simulink model "MIMO_FIXED"  (R2017a)
settings: Solver=VariableStepAuto  StartTime=0.0  StopTime=1000  RelTol=1e-3
libraries: dspsigops x80, commchan3 x4, commdigbbndpm3 x2, commfilt2 x2, commsink2 x1, commutil2 x1
(part 1 of 6)
settings Model: Creator=pc1  LastModifiedBy=U3
settings DataIOCC: SaveOutput=off  SignalLogging=off  DSMLogging=off  SaveTime=off
settings DebuggingCC: UnconnectedInputMsg=none  UnconnectedOutputMsg=none  UnconnectedLineMsg=none
settings SFSimCC: SimUseLocalCustomCode=on
settings RTWCC: RTWUseLocalCustomCode=on

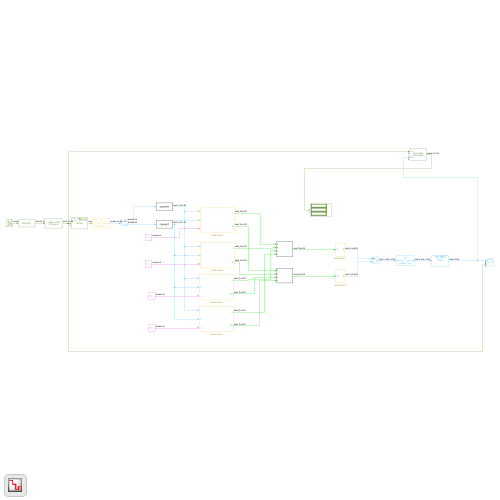
[thumbnail: Simulink's stored preview of the top-level diagram]
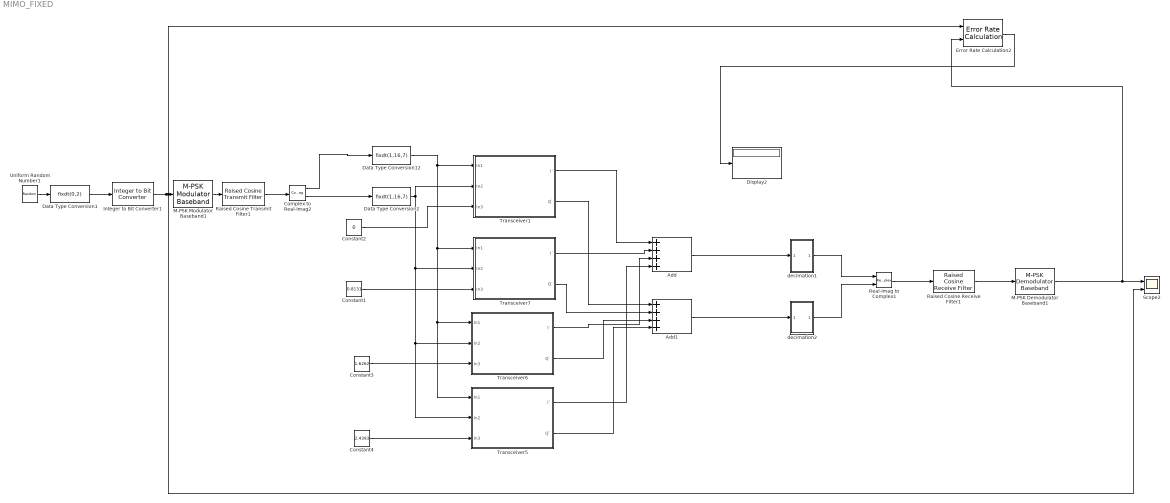
== system MIMO_FIXED ==
  Add : Sum  Inputs=++++  OutDataTypeStr=fixdt(1,8,4)
  Add1 : Sum  Inputs=++++  OutDataTypeStr=fixdt(1,8,4)
  Complex to Real-Imag2 : ComplexToRealImag
  Constant1 : Constant  Value=0.8131
  Constant2 : Constant  Value=0
  Constant3 : Constant  Value=1.6262
  Constant4 : Constant  Value=2.4393
  Data Type Conversion1 : DataTypeConversion  OutMin=0  OutMax=3  OutDataTypeStr=fixdt(0,2)  RndMeth=Round
  Data Type Conversion12 : DataTypeConversion  OutDataTypeStr=fixdt(1,16,7)  SaturateOnIntegerOverflow=on
  Data Type Conversion2 : DataTypeConversion  OutDataTypeStr=fixdt(1,16,7)  SaturateOnIntegerOverflow=on
  Display2 : Display
  Error Rate Calculation2 : commsink2/Error Rate Calculation  N=28  st_delay=0  cp_mode=Entire frame  subframe=[]  PMode=Port  WsName=ErrorVec  RsMode2=off  stop=off  numErr=100  maxBits=1e6
  Integer to Bit Converter1 : commutil2/Integer to Bit Converter  nbits=2  signedInputValues=Unsigned  bitOrder=MSB first  outDtype=Inherit via internal rule
  M-PSK Demodulator Baseband1 : commdigbbndpm3/M-PSK Demodulator Baseband  M=4  OutType=Bit  DecType=Hard decision  VarSource=Dialog  Variance=1  Dec=Gray  Mapping=[0:7]  Ph=pi/4  outDtype1=Inherit via internal rule  outDtype2=Inherit via internal rule  derotateFactorWordLen=16  derotateFactorDataTypeStr=Inherit: Same word length as input  derotateFactorLastDataTypeStr=Inherit: Same word length as input
  M-PSK Modulator Baseband1 : commdigbbndpm3/M-PSK Modulator Baseband  M=4  InType=Bit  Enc=Gray  Mapping=[0:7]  Ph=pi/4  outDtype=double  outWordLen=16  outUDDataType=sfix(16)  outFracLenMode=Best precision  outFracLen=15  outDataTypeStr=double  outLastDataTypeStr=double
  Raised Cosine Receive Filter1 : commfilt2/Raised Cosine Receive Filter  filtType=Square root  R=0.35  filtSpan=8  N=2  downFactor=1  downOffset=0  filterGain=22  InputProcessing=Columns as channels (frame based)  RateOptions=Allow multirate processing  framing=Mute  checkCoeff=off  variableName=rcRxFilt1  currentFiltSpan=8  D=(8)/2  inputOffset=0  sampMode=Mute  saveAsFlag=0  rateMode=Downsampling  checkGain=Normalized  launchFVT=on  roundingMode=Floor  overflowMode=off  coeffDataTypeStr=Inherit: Same word length as input  coeffMin=[]  coeffMax=[]  coeffLastDataTypeStr=Inherit: Same word length as input  accumDataTypeStr=Inherit: Same as product output  accumLastDataTypeStr=Inherit: Same as product output  outputDataTypeStr=Inherit: Same as accumulator  outputMin=[]  outputMax=[]  outputLastDataTypeStr=Inherit: Same as accumulator
  Raised Cosine Transmit Filter1 : commfilt2/Raised Cosine Transmit Filter  filtType=Square root  R=0.35  filtSpan=8  N=2  filterGain=22  InputProcessing=Columns as channels (frame based)  RateOptions=Allow multirate processing  framing=Mute  checkCoeff=off  variableName=rcTxFilt1  checkGain=Normalized  sampMode=Mute  saveAsFlag=0  currentFiltSpan=8  D=(8)/2  launchFVT=on  roundingMode=Floor  overflowMode=off  coeffDataTypeStr=Inherit: Same word length as input  coeffMin=[]  coeffMax=[]  coeffLastDataTypeStr=Inherit: Same word length as input  outputDataTypeStr=Inherit: Same as accumulator  outputMin=[]  outputMax=[]  outputLastDataTypeStr=Inherit: Same as accumulator
  Real-Imag to Complex1 : RealImagToComplex
  Scope2 : Scope  NumInputPorts=2
  Transceiver1 : Subsystem
  Transceiver5 : Subsystem
  Transceiver6 : Subsystem
  Transceiver7 : Subsystem
  Uniform Random Number1 : UniformRandomNumber  Minimum=0  Maximum=3  Seed=70  SampleTime=0.64
  decimation1 : Subsystem
  decimation2 : Subsystem
  wires:
  decimation1/1(Out1) -> Real-Imag to Complex1/1
  Complex to Real-Imag2/1 -> Data Type Conversion12/1
  Transceiver1/1(I`) -> Add/1
  Raised Cosine Transmit Filter1/1 -> Complex to Real-Imag2/1
  Error Rate Calculation2/1 -> Display2/1
  Raised Cosine Receive Filter1/1 -> M-PSK Demodulator Baseband1/1
  M-PSK Modulator Baseband1/1 -> Raised Cosine Transmit Filter1/1
  M-PSK Demodulator Baseband1/1 -> Scope2/1, Error Rate Calculation2/2
  Data Type Conversion1/1 -> Integer to Bit Converter1/1
  Integer to Bit Converter1/1 -> Error Rate Calculation2/1, Scope2/2, M-PSK Modulator Baseband1/1
  Real-Imag to Complex1/1 -> Raised Cosine Receive Filter1/1
  Uniform Random Number1/1 -> Data Type Conversion1/1
  Transceiver7/1(I`) -> Add/2
  Transceiver6/1(I`) -> Add/3
  Transceiver5/1(I`) -> Add/4
  Transceiver1/2(Q`) -> Add1/1
  Transceiver7/2(Q`) -> Add1/2
  Transceiver6/2(Q`) -> Add1/3
  Transceiver5/2(Q`) -> Add1/4
  Add1/1 -> decimation2/1(In1)
  Add/1 -> decimation1/1(In1)
  Complex to Real-Imag2/2 -> Data Type Conversion2/1
  Data Type Conversion12/1 -> Transceiver1/1(In1), Transceiver7/1(In1), Transceiver5/1(In1), Transceiver6/1(In1)
  Data Type Conversion2/1 -> Transceiver1/2(In2), Transceiver7/2(In2), Transceiver5/2(In2), Transceiver6/2(In2)
  Constant2/1 -> Transceiver1/3(In3)
  Constant1/1 -> Transceiver7/3(In3)
  Constant3/1 -> Transceiver6/3(In3)
  Constant4/1 -> Transceiver5/3(In3)
  decimation2/1(Out1) -> Real-Imag to Complex1/2

== system MIMO_FIXED/Transceiver1 ==
  In1 : Inport
  In2 : Inport  Port=2
  In3 : Inport  Port=3
  ADC 1 : Subsystem
  AWGN Channel : commchan3/AWGN Channel  InputProcessing=Columns as channels (frame based)  noiseMode="Signal to noise ratio  (SNR)"  EbNodB=10  EsNodB=10  SNRdB=22  bitsPerSym=1  Ps=1  Tsym=(1.000000e-02 * 1)  variance=0.0001  seed=67
  CWM_RX2 : Subsystem
  CWM_TX_Chain_1 : Subsystem
  DDC2 : Subsystem
  DUC2 : Subsystem
  Data Type Conversion : DataTypeConversion  OutDataTypeStr=fixdt(1,6,0)
  Data Type Conversion1 : DataTypeConversion  OutDataTypeStr=fixdt(1,6,0)
  Data Type Conversion2 : DataTypeConversion  OutDataTypeStr=fixdt(1,11,5)  RndMeth=Round  SaturateOnIntegerOverflow=on
  Data Type Conversion3 : DataTypeConversion  OutDataTypeStr=double  RndMeth=Round
  Data Type Conversion4 : DataTypeConversion  OutDataTypeStr=boolean  RndMeth=Round  SaturateOnIntegerOverflow=on
  Data Type Conversion7 : DataTypeConversion  OutDataTypeStr=fixdt(1,11,5)  RndMeth=Round  SaturateOnIntegerOverflow=on
  Gain : Gain  Gain=1/32
  Gain1 : Gain  Gain=1/256
  Gain2 : Gain  Gain=1/256
  Inter_Lever2 : Subsystem
  Interpolation 1 : Subsystem
  Interpolation 2 : Subsystem
  Subsystem1 : Subsystem
  Subsystem2 : Subsystem
  I` : Outport
  Q` : Outport  Port=2
  wires:
  Inter_Lever2/2(EVEN_Q) -> DDC2/2(EVEN_Q)
  DUC2/1(Out2) -> Gain/1
  AWGN Channel/1 -> ADC 1/1(In1)
  In3/1 -> CWM_TX_Chain_1/1(PHI), CWM_RX2/1(In1)
  Gain/1 -> Data Type Conversion3/1
  Inter_Lever2/1(ODD_I) -> DDC2/1(ODD_I)
  ADC 1/1(bits 1&0) -> Data Type Conversion4/1
  CWM_RX2/1(I`) -> I`/1
  DDC2/1(I_DDC) -> CWM_RX2/2(I_DDC)
  DDC2/2(Q_DDC) -> CWM_RX2/3(Q_DDC)
  In1/1 -> CWM_TX_Chain_1/2(Processor_I)
  In2/1 -> CWM_TX_Chain_1/3(Processor_Q)
  Subsystem2/1(Out1) -> Data Type Conversion/1
  Gain2/1 -> Data Type Conversion2/1
  CWM_RX2/2(Q`) -> Q`/1
  Data Type Conversion4/1 -> Inter_Lever2/1(bits 1&0)
  CWM_TX_Chain_1/2(Q_1) -> Interpolation 2/1(Input)
  Interpolation 1/1(Out1) -> Gain1/1
  Interpolation 2/1(Out1) -> Gain2/1
  Gain1/1 -> Data Type Conversion7/1
  Data Type Conversion7/1 -> Subsystem2/1(In1)
  Data Type Conversion2/1 -> Subsystem1/1(In1)
  Data Type Conversion1/1 -> DUC2/2(Q_1)
  Data Type Conversion/1 -> DUC2/1(I_1)
  Data Type Conversion3/1 -> AWGN Channel/1
  CWM_TX_Chain_1/1(I_1) -> Interpolation 1/1(Input)
  Subsystem1/1(Out1) -> Data Type Conversion1/1

== system MIMO_FIXED/Transceiver5 ==
  In1 : Inport
  In2 : Inport  Port=2
  In3 : Inport  Port=3
  ADC 1 : Subsystem
  AWGN Channel : commchan3/AWGN Channel  InputProcessing=Columns as channels (frame based)  noiseMode="Signal to noise ratio  (SNR)"  EbNodB=10  EsNodB=10  SNRdB=22  bitsPerSym=1  Ps=1  Tsym=(1.000000e-02 * 1)  variance=0.0001  seed=67
  CWM_RX2 : Subsystem
  CWM_TX_Chain_1 : Subsystem
  DDC2 : Subsystem
  DUC2 : Subsystem
  Data Type Conversion : DataTypeConversion  OutDataTypeStr=fixdt(1,6,0)
  Data Type Conversion1 : DataTypeConversion  OutDataTypeStr=fixdt(1,6,0)
  Data Type Conversion2 : DataTypeConversion  OutDataTypeStr=fixdt(1,11,5)  RndMeth=Round  SaturateOnIntegerOverflow=on
  Data Type Conversion3 : DataTypeConversion  OutDataTypeStr=double  RndMeth=Round
  Data Type Conversion4 : DataTypeConversion  OutDataTypeStr=boolean  RndMeth=Round  SaturateOnIntegerOverflow=on
  Data Type Conversion7 : DataTypeConversion  OutDataTypeStr=fixdt(1,11,5)  RndMeth=Round  SaturateOnIntegerOverflow=on
  Gain : Gain  Gain=1/32
  Gain1 : Gain  Gain=1/256
  Gain2 : Gain  Gain=1/256
  Inter_Lever2 : Subsystem
  Interpolation 1 : Subsystem
  Interpolation 2 : Subsystem
  Subsystem1 : Subsystem
  Subsystem2 : Subsystem
  I` : Outport
  Q` : Outport  Port=2
  wires:
  Inter_Lever2/2(EVEN_Q) -> DDC2/2(EVEN_Q)
  DUC2/1(Out2) -> Gain/1
  AWGN Channel/1 -> ADC 1/1(In1)
  In3/1 -> CWM_RX2/1(In1), CWM_TX_Chain_1/1(PHI)
  Gain/1 -> Data Type Conversion3/1
  Inter_Lever2/1(ODD_I) -> DDC2/1(ODD_I)
  ADC 1/1(bits 1&0) -> Data Type Conversion4/1
  CWM_RX2/1(I`) -> I`/1
  DDC2/1(I_DDC) -> CWM_RX2/2(I_DDC)
  DDC2/2(Q_DDC) -> CWM_RX2/3(Q_DDC)
  In1/1 -> CWM_TX_Chain_1/2(Processor_I)
  In2/1 -> CWM_TX_Chain_1/3(Processor_Q)
  Subsystem2/1(Out1) -> Data Type Conversion/1
  Gain2/1 -> Data Type Conversion2/1
  CWM_RX2/2(Q`) -> Q`/1
  Data Type Conversion4/1 -> Inter_Lever2/1(bits 1&0)
  CWM_TX_Chain_1/2(Q_1) -> Interpolation 2/1(Input)
  Interpolation 1/1(Out1) -> Gain1/1
  Interpolation 2/1(Out1) -> Gain2/1
  Gain1/1 -> Data Type Conversion7/1
  Data Type Conversion7/1 -> Subsystem2/1(In1)
  Data Type Conversion2/1 -> Subsystem1/1(In1)
  Data Type Conversion1/1 -> DUC2/2(Q_1)
  Data Type Conversion/1 -> DUC2/1(I_1)
  Data Type Conversion3/1 -> AWGN Channel/1
  CWM_TX_Chain_1/1(I_1) -> Interpolation 1/1(Input)
  Subsystem1/1(Out1) -> Data Type Conversion1/1

== system MIMO_FIXED/Transceiver6 ==
  In1 : Inport
  In2 : Inport  Port=2
  In3 : Inport  Port=3
  ADC 1 : Subsystem
  AWGN Channel : commchan3/AWGN Channel  InputProcessing=Columns as channels (frame based)  noiseMode="Signal to noise ratio  (SNR)"  EbNodB=10  EsNodB=10  SNRdB=22  bitsPerSym=1  Ps=1  Tsym=(1.000000e-02 * 1)  variance=0.0001  seed=67
  CWM_RX2 : Subsystem
  CWM_TX_Chain_1 : Subsystem
  DDC2 : Subsystem
  DUC2 : Subsystem
  Data Type Conversion : DataTypeConversion  OutDataTypeStr=fixdt(1,6,0)
  Data Type Conversion1 : DataTypeConversion  OutDataTypeStr=fixdt(1,6,0)
  Data Type Conversion2 : DataTypeConversion  OutDataTypeStr=fixdt(1,11,5)  RndMeth=Round  SaturateOnIntegerOverflow=on
  Data Type Conversion3 : DataTypeConversion  OutDataTypeStr=double  RndMeth=Round
  Data Type Conversion4 : DataTypeConversion  OutDataTypeStr=boolean  RndMeth=Round  SaturateOnIntegerOverflow=on
  Data Type Conversion7 : DataTypeConversion  OutDataTypeStr=fixdt(1,11,5)  RndMeth=Round  SaturateOnIntegerOverflow=on
  Gain : Gain  Gain=1/32
  Gain1 : Gain  Gain=1/256
  Gain2 : Gain  Gain=1/256
  Inter_Lever2 : Subsystem
  Interpolation 1 : Subsystem
  Interpolation 2 : Subsystem
  Subsystem1 : Subsystem
  Subsystem2 : Subsystem
  I` : Outport
  Q` : Outport  Port=2
  wires:
  Inter_Lever2/2(EVEN_Q) -> DDC2/2(EVEN_Q)
  DUC2/1(Out2) -> Gain/1
  AWGN Channel/1 -> ADC 1/1(In1)
  In3/1 -> CWM_RX2/1(In1), CWM_TX_Chain_1/1(PHI)
  Gain/1 -> Data Type Conversion3/1
  Inter_Lever2/1(ODD_I) -> DDC2/1(ODD_I)
  ADC 1/1(bits 1&0) -> Data Type Conversion4/1
  CWM_RX2/1(I`) -> I`/1
  DDC2/1(I_DDC) -> CWM_RX2/2(I_DDC)
  DDC2/2(Q_DDC) -> CWM_RX2/3(Q_DDC)
  In1/1 -> CWM_TX_Chain_1/2(Processor_I)
  In2/1 -> CWM_TX_Chain_1/3(Processor_Q)
  Subsystem2/1(Out1) -> Data Type Conversion/1
  Gain2/1 -> Data Type Conversion2/1
  CWM_RX2/2(Q`) -> Q`/1
  Data Type Conversion4/1 -> Inter_Lever2/1(bits 1&0)
  CWM_TX_Chain_1/2(Q_1) -> Interpolation 2/1(Input)
  Interpolation 1/1(Out1) -> Gain1/1
  Interpolation 2/1(Out1) -> Gain2/1
  Gain1/1 -> Data Type Conversion7/1
  Data Type Conversion7/1 -> Subsystem2/1(In1)
  Data Type Conversion2/1 -> Subsystem1/1(In1)
  Data Type Conversion1/1 -> DUC2/2(Q_1)
  Data Type Conversion/1 -> DUC2/1(I_1)
  Data Type Conversion3/1 -> AWGN Channel/1
  CWM_TX_Chain_1/1(I_1) -> Interpolation 1/1(Input)
  Subsystem1/1(Out1) -> Data Type Conversion1/1

== system MIMO_FIXED/Transceiver7 ==
  In1 : Inport
  In2 : Inport  Port=2
  In3 : Inport  Port=3
  ADC 1 : Subsystem
  AWGN Channel : commchan3/AWGN Channel  InputProcessing=Columns as channels (frame based)  noiseMode="Signal to noise ratio  (SNR)"  EbNodB=10  EsNodB=10  SNRdB=22  bitsPerSym=1  Ps=1  Tsym=(1.000000e-02 * 1)  variance=0.0001  seed=67
  CWM_RX2 : Subsystem
  CWM_TX_Chain_1 : Subsystem
  DDC2 : Subsystem
  DUC2 : Subsystem
  Data Type Conversion : DataTypeConversion  OutDataTypeStr=fixdt(1,6,0)
  Data Type Conversion1 : DataTypeConversion  OutDataTypeStr=fixdt(1,6,0)
  Data Type Conversion2 : DataTypeConversion  OutDataTypeStr=fixdt(1,11,5)  RndMeth=Round  SaturateOnIntegerOverflow=on
  Data Type Conversion3 : DataTypeConversion  OutDataTypeStr=double  RndMeth=Round
  Data Type Conversion4 : DataTypeConversion  OutDataTypeStr=boolean  RndMeth=Round  SaturateOnIntegerOverflow=on
  Data Type Conversion7 : DataTypeConversion  OutDataTypeStr=fixdt(1,11,5)  RndMeth=Round  SaturateOnIntegerOverflow=on
  Gain : Gain  Gain=1/32
  Gain1 : Gain  Gain=1/256
  Gain2 : Gain  Gain=1/256
  Inter_Lever2 : Subsystem
  Interpolation 1 : Subsystem
  Interpolation 2 : Subsystem
  Subsystem1 : Subsystem
  Subsystem2 : Subsystem
  I` : Outport
  Q` : Outport  Port=2
  wires:
  Inter_Lever2/2(EVEN_Q) -> DDC2/2(EVEN_Q)
  DUC2/1(Out2) -> Gain/1
  AWGN Channel/1 -> ADC 1/1(In1)
  In3/1 -> CWM_RX2/1(In1), CWM_TX_Chain_1/1(PHI)
  Gain/1 -> Data Type Conversion3/1
  Inter_Lever2/1(ODD_I) -> DDC2/1(ODD_I)
  ADC 1/1(bits 1&0) -> Data Type Conversion4/1
  CWM_RX2/1(I`) -> I`/1
  DDC2/1(I_DDC) -> CWM_RX2/2(I_DDC)
  DDC2/2(Q_DDC) -> CWM_RX2/3(Q_DDC)
  In1/1 -> CWM_TX_Chain_1/2(Processor_I)
  In2/1 -> CWM_TX_Chain_1/3(Processor_Q)
  Subsystem2/1(Out1) -> Data Type Conversion/1
  Gain2/1 -> Data Type Conversion2/1
  CWM_RX2/2(Q`) -> Q`/1
  Data Type Conversion4/1 -> Inter_Lever2/1(bits 1&0)
  CWM_TX_Chain_1/2(Q_1) -> Interpolation 2/1(Input)
  Interpolation 1/1(Out1) -> Gain1/1
  Interpolation 2/1(Out1) -> Gain2/1
  Gain1/1 -> Data Type Conversion7/1
  Data Type Conversion7/1 -> Subsystem2/1(In1)
  Data Type Conversion2/1 -> Subsystem1/1(In1)
  Data Type Conversion1/1 -> DUC2/2(Q_1)
  Data Type Conversion/1 -> DUC2/1(I_1)
  Data Type Conversion3/1 -> AWGN Channel/1
  CWM_TX_Chain_1/1(I_1) -> Interpolation 1/1(Input)
  Subsystem1/1(Out1) -> Data Type Conversion1/1

== system MIMO_FIXED/decimation1 ==
  In1 : Inport
  Add1 : Sum  OutDataTypeStr=fixdt(1,19,0)
  Data Type Conversion12 : DataTypeConversion  OutDataTypeStr=fixdt(1,16,4)  SaturateOnIntegerOverflow=on
  Data Type Conversion9 : DataTypeConversion  OutDataTypeStr=fixdt(1,12,4)  SaturateOnIntegerOverflow=on
  Delay{7..10,12..15} (8 alike) : Delay  DelayLength=1
  Downsample{,1..3,6..9} (8 alike) : DownSample  N=8  RateOptions=Allow multirate processing
  Downsample4 : DownSample  RateOptions=Allow multirate processing
  Downsample5 : DownSample  RateOptions=Allow multirate processing
  E0(Z) : Subsystem
  E1(Z) : Subsystem
  E10 : Subsystem
  E11 : Subsystem
  E12 : Subsystem
  E13 : Subsystem
  E14 : Subsystem
  E15 : Subsystem
  E8 : Subsystem
  E9 : Subsystem
  Gain : Gain  Gain=16
  Gain1 : Gain  Gain=1/128
  Gain2 : Gain  Gain=1/16
  Gain4 : Gain  Gain=1/512
  Gain5 : Gain  Gain=1/16
  Gain6 : Gain  Gain=16
  Sum3 : Sum  Inputs=|++++++++
  To Workspace2 : ToWorkspace  VariableName=simout2  SampleTime=-1
      settings: Save2DSignal=2-D array (concatenate along first dimension)
  To Workspace3 : ToWorkspace  VariableName=simout3  SampleTime=-1
      settings: Save2DSignal=2-D array (concatenate along first dimension)
  Out1 : Outport
  wires:
  Gain1/1 -> Data Type Conversion9/1
  Downsample9/1 -> E15/1(In1)
  E12/1(Out1) -> Sum3/5
  Downsample1/1 -> E9/1(In1)
  Downsample7/1 -> E13/1(In1)
  Delay8/1 -> Delay9/1, Downsample2/1
  Downsample2/1 -> E10/1(In1)
  Downsample6/1 -> E12/1(In1)
  E15/1(Out1) -> Sum3/8
  E14/1(Out1) -> Sum3/7
  Delay13/1 -> Delay14/1, Downsample7/1
  Delay7/1 -> Delay8/1, Downsample1/1
  Downsample8/1 -> E14/1(In1)
  Delay12/1 -> Delay13/1, Downsample6/1
  E11/1(Out1) -> Sum3/4
  Downsample/1 -> E8/1(In1)
  E9/1(Out1) -> Sum3/2
  E8/1(Out1) -> Sum3/1
  Delay14/1 -> Delay15/1, Downsample8/1
  E13/1(Out1) -> Sum3/6
  E10/1(Out1) -> Sum3/3
  Delay15/1 -> Downsample9/1
  Downsample3/1 -> E11/1(In1)
  In1/1 -> Gain/1
  Delay9/1 -> Delay12/1, Downsample3/1
  Gain/1 -> Delay7/1, Downsample/1
  Gain2/1 -> Gain1/1
  Sum3/1 -> Gain2/1
  Data Type Conversion12/1 -> Out1/1
  Gain5/1 -> Gain4/1
  Data Type Conversion9/1 -> Gain6/1
  Gain4/1 -> Data Type Conversion12/1
  Add1/1 -> To Workspace3/1, Gain5/1
  Gain6/1 -> To Workspace2/1, Downsample4/1, Delay10/1
  E0(Z)/1(Out1) -> Add1/1
  Delay10/1 -> Downsample5/1
  Downsample4/1 -> E0(Z)/1(Input)
  Downsample5/1 -> E1(Z)/1(Input1)
  E1(Z)/1(Output) -> Add1/2

== system MIMO_FIXED/decimation2 ==
  In1 : Inport
  Add1 : Sum  OutDataTypeStr=fixdt(1,19,0)
  Data Type Conversion12 : DataTypeConversion  OutDataTypeStr=fixdt(1,16,4)  SaturateOnIntegerOverflow=on
  Data Type Conversion9 : DataTypeConversion  OutDataTypeStr=fixdt(1,12,4)  SaturateOnIntegerOverflow=on
  Delay{7..10,12..15} (8 alike) : Delay  DelayLength=1
  Downsample{,1..3,6..9} (8 alike) : DownSample  N=8  RateOptions=Allow multirate processing
  Downsample4 : DownSample  RateOptions=Allow multirate processing
  Downsample5 : DownSample  RateOptions=Allow multirate processing
  E0(Z) : Subsystem
  E1(Z) : Subsystem
  E10 : Subsystem
  E11 : Subsystem
  E12 : Subsystem
  E13 : Subsystem
  E14 : Subsystem
  E15 : Subsystem
  E8 : Subsystem
  E9 : Subsystem
  Gain : Gain  Gain=16
  Gain1 : Gain  Gain=1/128
  Gain2 : Gain  Gain=1/16
  Gain4 : Gain  Gain=1/512
  Gain5 : Gain  Gain=1/16
  Gain6 : Gain  Gain=16
  Sum3 : Sum  Inputs=|++++++++
  To Workspace1 : ToWorkspace  VariableName=simout1  SampleTime=-1
      settings: Save2DSignal=2-D array (concatenate along first dimension)
  Out1 : Outport
  wires:
  Gain1/1 -> Data Type Conversion9/1
  Downsample9/1 -> E15/1(In1)
  E12/1(Out1) -> Sum3/5
  Downsample1/1 -> E9/1(In1)
  Downsample7/1 -> E13/1(In1)
  Delay8/1 -> Delay9/1, Downsample2/1
  Downsample2/1 -> E10/1(In1)
  Downsample6/1 -> E12/1(In1)
  E15/1(Out1) -> Sum3/8
  E14/1(Out1) -> Sum3/7
  Delay13/1 -> Delay14/1, Downsample7/1
  Delay7/1 -> Delay8/1, Downsample1/1
  Downsample8/1 -> E14/1(In1)
  Delay12/1 -> Delay13/1, Downsample6/1
  E11/1(Out1) -> Sum3/4
  Downsample/1 -> E8/1(In1)
  E9/1(Out1) -> Sum3/2
  E8/1(Out1) -> Sum3/1
  Delay14/1 -> Delay15/1, Downsample8/1
  E13/1(Out1) -> Sum3/6
  E10/1(Out1) -> Sum3/3
  Delay15/1 -> Downsample9/1
  Downsample3/1 -> E11/1(In1)
  In1/1 -> Gain/1
  Delay9/1 -> Delay12/1, Downsample3/1
  Gain/1 -> Delay7/1, Downsample/1
  Gain2/1 -> Gain1/1
  Sum3/1 -> Gain2/1
  Data Type Conversion12/1 -> Out1/1
  Gain5/1 -> Gain4/1
  Data Type Conversion9/1 -> Gain6/1
  Gain4/1 -> Data Type Conversion12/1
  Add1/1 -> Gain5/1
  Gain6/1 -> Downsample4/1, Delay10/1
  E0(Z)/1(Out1) -> Add1/1
  Delay10/1 -> Downsample5/1
  Downsample4/1 -> E0(Z)/1(Input)
  Downsample5/1 -> E1(Z)/1(Input1)
  E1(Z)/1(Output) -> To Workspace1/1, Add1/2

== system MIMO_FIXED/Transceiver1/ADC 1 ==
  In1 : Inport
  SigmaDelta ADC : Subsystem
  Switch : Switch  Criteria=u2 > Threshold  OutDataTypeStr=boolean
  Zero : Constant  Value=0
  bits 1&0 : Outport
  wires:
  SigmaDelta ADC/1(Out) -> Switch/1, Switch/2
  Zero/1 -> Switch/3
  In1/1 -> SigmaDelta ADC/1(In)
  Switch/1 -> bits 1&0/1

== system MIMO_FIXED/Transceiver1/CWM_RX2 ==
  In1 : Inport
  I_DDC : Inport  Port=2
  Q_DDC : Inport  Port=3
  Add : Sum
  Add1 : Sum  Inputs=-+
  Data Type Conversion{,1..9} (10 alike) : DataTypeConversion  OutDataTypeStr=fixdt(1,6,4)  SaturateOnIntegerOverflow=on
  Gain{,2,4,6} (4 alike) : Gain  Gain=-1
  Gain{1,3,5,7} (4 alike) : Gain
  Multiport Switch{,1,4..5} (4 alike) : MultiPortSwitch  DataPortOrder=Zero-based contiguous  Inputs=2  zeroidx=on  RndMeth=Nearest
  Trigonometric Function{,1,4..5} (4 alike) : Trigonometry
  Trigonometric Function{2..3,6..7} (4 alike) : Trigonometry  Operator=cos
  I` : Outport
  Q` : Outport  Port=2
  wires:
  Multiport Switch/1 -> Add1/1
  Add/1 -> Data Type Conversion8/1
  I_DDC/1 -> Multiport Switch1/1, Multiport Switch/1
  Gain2/1 -> Data Type Conversion6/1
  Trigonometric Function5/1 -> Gain5/1
  Data Type Conversion6/1 -> Multiport Switch1/2
  Data Type Conversion7/1 -> Multiport Switch/3
  Gain5/1 -> Data Type Conversion3/1
  Gain4/1 -> Data Type Conversion4/1
  Trigonometric Function1/1 -> Gain1/1
  Data Type Conversion2/1 -> Multiport Switch5/2
  Gain1/1 -> Data Type Conversion7/1
  Gain3/1 -> Data Type Conversion5/1
  Trigonometric Function3/1 -> Gain3/1
  Add1/1 -> Data Type Conversion9/1
  Gain/1 -> Data Type Conversion/1
  Trigonometric Function2/1 -> Gain2/1
  In1/1 -> Trigonometric Function3/1, Trigonometric Function6/1, Trigonometric Function7/1, Trigonometric Function5/1, Trigonometric Function4/1, Trigonometric Function2/1, Trigonometric Function1/1, Trigonometric Function/1
  Q_DDC/1 -> Multiport Switch5/1, Multiport Switch4/1
  Data Type Conversion1/1 -> Multiport Switch5/3
  Data Type Conversion4/1 -> Multiport Switch4/2
  Trigonometric Function6/1 -> Gain6/1
  Gain7/1 -> Data Type Conversion1/1
  Trigonometric Function4/1 -> Gain4/1
  Trigonometric Function/1 -> Gain/1
  Multiport Switch1/1 -> Add/1
  Multiport Switch4/1 -> Add/2
  Trigonometric Function7/1 -> Gain7/1
  Multiport Switch5/1 -> Add1/2
  Data Type Conversion3/1 -> Multiport Switch4/3
  Gain6/1 -> Data Type Conversion2/1
  Data Type Conversion/1 -> Multiport Switch/2
  Data Type Conversion5/1 -> Multiport Switch1/3
  Data Type Conversion8/1 -> I`/1
  Data Type Conversion9/1 -> Q`/1

== system MIMO_FIXED/Transceiver1/CWM_TX_Chain_1 ==
  PHI : Inport
  Processor_I : Inport  Port=2
  Processor_Q : Inport  Port=3
  Add : Sum  OutDataTypeStr=double  RndMeth=Round  SaturateOnIntegerOverflow=on
  Add1 : Sum  OutDataTypeStr=double
  Data Type Conversion : DataTypeConversion  OutDataTypeStr=fixdt(1,6,4)  SaturateOnIntegerOverflow=on
  Data Type Conversion1 : DataTypeConversion  OutDataTypeStr=fixdt(1,6,4)  RndMeth=Round  SaturateOnIntegerOverflow=on
  Data Type Conversion12 : DataTypeConversion  OutDataTypeStr=fixdt(1,16,9)  SaturateOnIntegerOverflow=on
  Data Type Conversion2 : DataTypeConversion  OutDataTypeStr=fixdt(1,6,4)  RndMeth=Round  SaturateOnIntegerOverflow=on
  Data Type Conversion3 : DataTypeConversion  OutDataTypeStr=fixdt(1,6,4)  SaturateOnIntegerOverflow=on
  Data Type Conversion4 : DataTypeConversion  OutDataTypeStr=fixdt(1,16,7)  SaturateOnIntegerOverflow=on
  Data Type Conversion5 : DataTypeConversion  OutDataTypeStr=fixdt(1,16,9)  SaturateOnIntegerOverflow=on
  Data Type Conversion6 : DataTypeConversion  OutDataTypeStr=fixdt(1,16,9)  SaturateOnIntegerOverflow=on
  Data Type Conversion7 : DataTypeConversion  OutDataTypeStr=fixdt(1,18,9)  SaturateOnIntegerOverflow=on
  Data Type Conversion8 : DataTypeConversion  OutDataTypeStr=fixdt(1,18,9)  SaturateOnIntegerOverflow=on
  Gain1 : Gain  Gain=-1
  Gain2 : Gain
  Gain3 : Gain
  Gain4 : Gain
  Product{,1..3} (4 alike) : Product
  Trigonometric Function1 : Trigonometry
  Trigonometric Function2 : Trigonometry  Operator=cos
  Trigonometric Function3 : Trigonometry  Operator=cos
  Trigonometric Function4 : Trigonometry
  I_1 : Outport
  Q_1 : Outport  Port=2
  wires:
  Trigonometric Function2/1 -> Gain2/1
  Gain2/1 -> Data Type Conversion/1
  Processor_Q/1 -> Product1/2, Product3/2
  Processor_I/1 -> Product2/1, Product/1
  Gain1/1 -> Data Type Conversion1/1
  Product/1 -> Data Type Conversion12/1
  Trigonometric Function1/1 -> Gain1/1
  PHI/1 -> Trigonometric Function2/1, Trigonometric Function1/1, Trigonometric Function4/1, Trigonometric Function3/1
  Data Type Conversion1/1 -> Product1/1
  Gain3/1 -> Data Type Conversion3/1
  Product2/1 -> Data Type Conversion5/1
  Data Type Conversion/1 -> Product/2
  Data Type Conversion2/1 -> Product2/2
  Data Type Conversion3/1 -> Product3/1
  Product3/1 -> Data Type Conversion6/1
  Trigonometric Function3/1 -> Gain3/1
  Product1/1 -> Data Type Conversion4/1
  Gain4/1 -> Data Type Conversion2/1
  Trigonometric Function4/1 -> Gain4/1
  Add1/1 -> Data Type Conversion8/1
  Data Type Conversion7/1 -> I_1/1
  Data Type Conversion8/1 -> Q_1/1
  Data Type Conversion12/1 -> Add/1
  Data Type Conversion4/1 -> Add/2
  Data Type Conversion5/1 -> Add1/1
  Data Type Conversion6/1 -> Add1/2
  Add/1 -> Data Type Conversion7/1

== system MIMO_FIXED/Transceiver1/DDC2 ==
  ODD_I : Inport
  EVEN_Q : Inport  Port=2
  Local_Oscilator1 : DiscretePulseGenerator  PhaseDelay=1  SampleTime=0.02
  Logical Operator : Logic  Operator=NXOR  AllPortsSameDT=off  OutDataTypeStr=boolean
  Logical Operator1 : Logic  Operator=NXOR  AllPortsSameDT=off  OutDataTypeStr=boolean
  NOT : Logic  Operator=NOT  IconShape=distinctive  AllPortsSameDT=off  OutDataTypeStr=boolean
  I_DDC : Outport
  Q_DDC : Outport  Port=2
  wires:
  Logical Operator/1 -> I_DDC/1
  EVEN_Q/1 -> Logical Operator1/2
  ODD_I/1 -> Logical Operator/1
  Logical Operator1/1 -> Q_DDC/1
  Local_Oscilator1/1 -> NOT/1
  NOT/1 -> Logical Operator1/1, Logical Operator/2

== system MIMO_FIXED/Transceiver1/DUC2 ==
  I_1 : Inport
  Q_1 : Inport  Port=2
  -cos : Sin  SineType=Sample based  Frequency=2*pi*100  Phase=pi/2  Samples=4  SampleTime=0.01  Offset=3
  -sin1 : Sin  SineType=Sample based  Frequency=(2*pi*100)/4  Samples=4  SampleTime=.01  Offset=2
  Add : Sum
  Constant : Constant  Value=0
  Constant1 : Constant  Value=0
  Data Type Conversion : DataTypeConversion  OutDataTypeStr=fixdt(1,2,0)  RndMeth=Round
  Data Type Conversion1 : DataTypeConversion  OutDataTypeStr=fixdt(1,2,0)  RndMeth=Round
  Data Type Conversion{2..3,5..6} (4 alike) : DataTypeConversion  OutDataTypeStr=fixdt(1,6,0)
  Data Type Conversion4 : DataTypeConversion  OutDataTypeStr=fixdt(1,7,0)
  Gain : Gain  Gain=-1
  Gain1 : Gain  Gain=-1
  Multiport Switch : MultiPortSwitch  DataPortOrder=Specify indices  DataPortIndices={1,0,-1}  RndMeth=Nearest
  Multiport Switch1 : MultiPortSwitch  DataPortOrder=Specify indices  DataPortIndices={1,0,-1}  RndMeth=Nearest
  Out2 : Outport
  wires:
  Constant/1 -> Multiport Switch1/3
  Q_1/1 -> Multiport Switch/2, Gain1/1
  I_1/1 -> Multiport Switch1/2, Gain/1
  Gain1/1 -> Data Type Conversion2/1
  -sin1/1 -> Data Type Conversion1/1
  -cos/1 -> Data Type Conversion/1
  Multiport Switch/1 -> Data Type Conversion5/1
  Add/1 -> Data Type Conversion4/1
  Multiport Switch1/1 -> Data Type Conversion6/1
  Constant1/1 -> Multiport Switch/3
  Gain/1 -> Data Type Conversion3/1
  Data Type Conversion/1 -> Multiport Switch1/1
  Data Type Conversion1/1 -> Multiport Switch/1
  Data Type Conversion2/1 -> Multiport Switch/4
  Data Type Conversion3/1 -> Multiport Switch1/4
  Data Type Conversion6/1 -> Add/1
  Data Type Conversion5/1 -> Add/2
  Data Type Conversion4/1 -> Out2/1

== system MIMO_FIXED/Transceiver1/Inter_Lever2 ==
  bits 1&0 : Inport
  Delay1 : Delay  DelayLength=1  InitialCondition=0
  Delay2 : Delay  DelayLength=1  InitialCondition=0
  Downsample : DownSample  RateOptions=Allow multirate processing
  Downsample1 : DownSample  RateOptions=Allow multirate processing
  ODD_I : Outport
  EVEN_Q : Outport  Port=2
  wires:
  Delay1/1 -> Downsample1/1
  Downsample/1 -> Delay2/1
  Downsample1/1 -> EVEN_Q/1
  bits 1&0/1 -> Delay1/1, Downsample/1
  Delay2/1 -> ODD_I/1

== system MIMO_FIXED/Transceiver1/Interpolation 1 ==
  Input : Inport
  Data Type Conversion2 : DataTypeConversion  OutDataTypeStr=fixdt(1,11,6)  SaturateOnIntegerOverflow=on
  Data Type Conversion5 : DataTypeConversion  OutDataTypeStr=fixdt(1,23,0)  SaturateOnIntegerOverflow=on
  Gain : Gain  Gain=512
  Gain1 : Gain  Gain=1/64
  Gain2 : Gain  Gain=1/512
  Gain3 : Gain  Gain=1/512
  Gain5 : Gain  Gain=64
  Half_band : Subsystem
  comb_filter : Subsystem
  Out1 : Outport
  wires:
  Input/1 -> Gain/1
  Gain5/1 -> comb_filter/1(In1)
  Gain1/1 -> Out1/1
  Data Type Conversion2/1 -> Gain5/1
  Gain2/1 -> Gain3/1
  Gain3/1 -> Data Type Conversion2/1
  Data Type Conversion5/1 -> Gain2/1
  Gain/1 -> Half_band/1(Input)
  Half_band/1(Out1) -> Data Type Conversion5/1
  comb_filter/1(Out1) -> Gain1/1

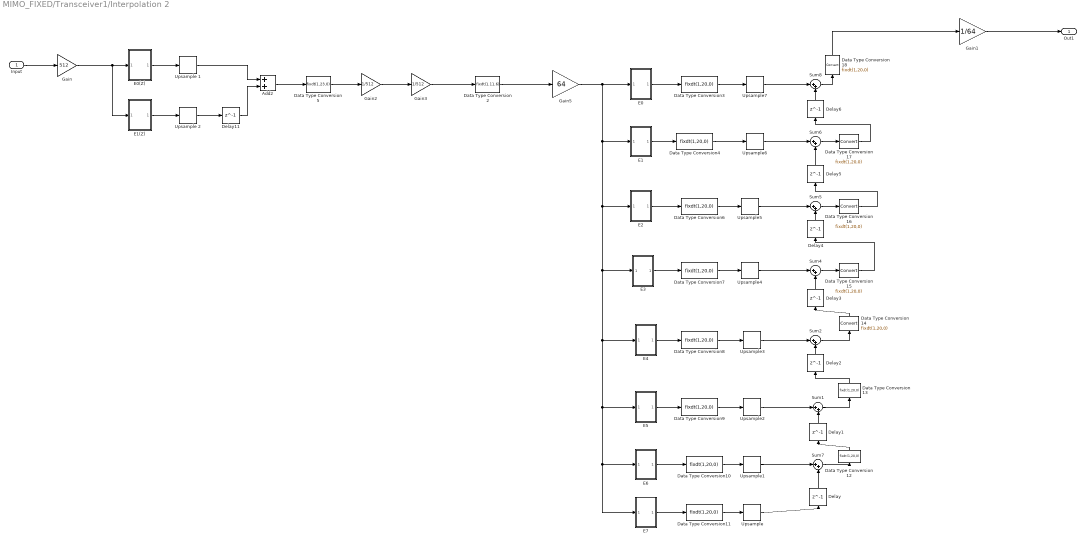
== system MIMO_FIXED/Transceiver1/Interpolation 2 ==
  Input : Inport
  Add2 : Sum
  Data Type Conversion{3..4,6..18} (15 alike) : DataTypeConversion  OutDataTypeStr=fixdt(1,20,0)  SaturateOnIntegerOverflow=on
  Data Type Conversion2 : DataTypeConversion  OutDataTypeStr=fixdt(1,11,6)  SaturateOnIntegerOverflow=on
  Data Type Conversion5 : DataTypeConversion  OutDataTypeStr=fixdt(1,23,0)  SaturateOnIntegerOverflow=on
  Delay{,1..6,11} (8 alike) : Delay  DelayLength=1
  E0 : Subsystem
  E0(Z) : Subsystem
  E1 : Subsystem
  E1(Z) : Subsystem
  E2 : Subsystem
  E3 : Subsystem
  E4 : Subsystem
  E5 : Subsystem
  E6 : Subsystem
  E7 : Subsystem
  Gain : Gain  Gain=512
  Gain1 : Gain  Gain=1/64
  Gain2 : Gain  Gain=1/512
  Gain3 : Gain  Gain=1/512
  Gain5 : Gain  Gain=64
  Sum{1..2,4..8} (7 alike) : Sum  Inputs=|++
  Upsample{,1..7} (8 alike) : dspsigops/Upsample  N=8  phase=0  RateOptions=Allow multirate processing  ic=0  mode=Unused parameter value
  Upsample 1 : dspsigops/Upsample  N=2  phase=0  RateOptions=Allow multirate processing  ic=0  mode=Unused parameter value
  Upsample 2 : dspsigops/Upsample  N=2  phase=0  RateOptions=Allow multirate processing  ic=0  mode=Unused parameter value
  Out1 : Outport
  wires:
  Upsample/1 -> Delay/1
  Delay5/1 -> Sum6/2
  Upsample6/1 -> Sum6/1
  Delay4/1 -> Sum5/2
  Delay3/1 -> Sum4/2
  Sum6/1 -> Data Type Conversion17/1
  Upsample1/1 -> Sum7/1
  Upsample2/1 -> Sum1/1
  Input/1 -> Gain/1
  Upsample 2/1 -> Delay11/1
  Delay6/1 -> Sum8/2
  E0/1(Out1) -> Data Type Conversion3/1
  Delay/1 -> Sum7/2
  E1/1(Out1) -> Data Type Conversion4/1
  Delay1/1 -> Sum1/2
  Sum5/1 -> Data Type Conversion16/1
  Sum4/1 -> Data Type Conversion15/1
  Upsample5/1 -> Sum5/1
  Upsample 1/1 -> Add2/1
  Upsample4/1 -> Sum4/1
  Delay11/1 -> Add2/2
  Sum2/1 -> Data Type Conversion14/1
  E3/1(Out1) -> Data Type Conversion7/1
  Delay2/1 -> Sum2/2
  Upsample7/1 -> Sum8/1
  Upsample3/1 -> Sum2/1
  E2/1(Out1) -> Data Type Conversion6/1
  E4/1(Out1) -> Data Type Conversion8/1
  E0(Z)/1(Out1) -> Upsample 1/1
  Data Type Conversion3/1 -> Upsample7/1
  Data Type Conversion4/1 -> Upsample6/1
  Data Type Conversion6/1 -> Upsample5/1
  Data Type Conversion7/1 -> Upsample4/1
  Data Type Conversion8/1 -> Upsample3/1
  Data Type Conversion9/1 -> Upsample2/1
  Data Type Conversion10/1 -> Upsample1/1
  Data Type Conversion11/1 -> Upsample/1
  Data Type Conversion12/1 -> Delay1/1
  Sum7/1 -> Data Type Conversion12/1
  Data Type Conversion13/1 -> Delay2/1
  Data Type Conversion14/1 -> Delay3/1
  Sum1/1 -> Data Type Conversion13/1
  Data Type Conversion15/1 -> Delay4/1
  Data Type Conversion16/1 -> Delay5/1
  Data Type Conversion17/1 -> Delay6/1
  Data Type Conversion18/1 -> Gain1/1
  Sum8/1 -> Data Type Conversion18/1
  E5/1(Out1) -> Data Type Conversion9/1
  E6/1(Out1) -> Data Type Conversion10/1
  E7/1(Out1) -> Data Type Conversion11/1
  Gain5/1 -> E0/1(In1), E7/1(In1), E6/1(In1), E5/1(In1), E4/1(In1), E3/1(In1), E2/1(In1), E1/1(In1)
  Gain1/1 -> Out1/1
  Gain/1 -> E0(Z)/1(Input), E1(Z)/1(Input1)
  Data Type Conversion2/1 -> Gain5/1
  Gain2/1 -> Gain3/1
  E1(Z)/1(Output) -> Upsample 2/1
  Gain3/1 -> Data Type Conversion2/1
  Add2/1 -> Data Type Conversion5/1
  Data Type Conversion5/1 -> Gain2/1

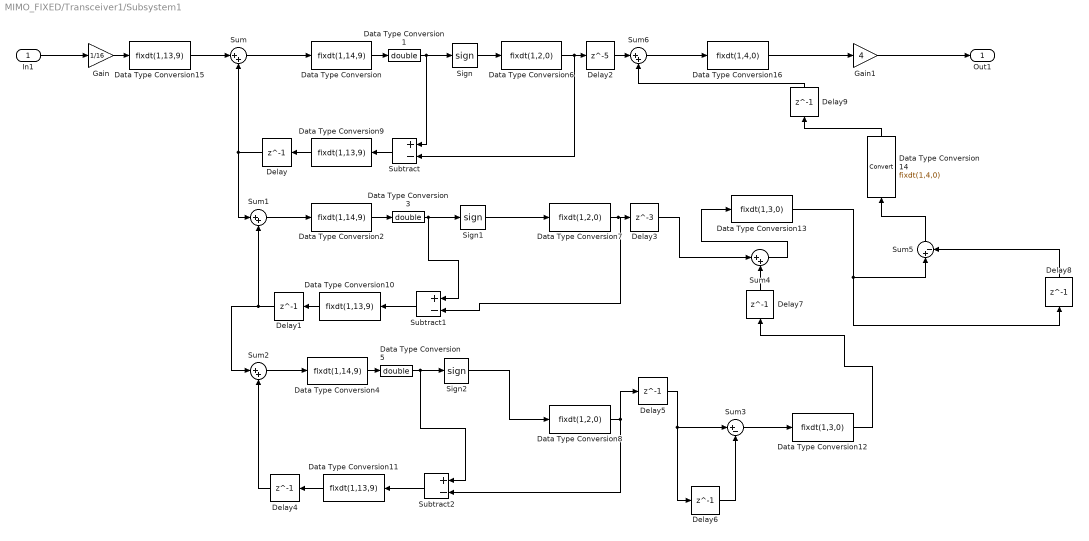
== system MIMO_FIXED/Transceiver1/Subsystem1 ==
  In1 : Inport
  Data Type Conversion : DataTypeConversion  OutDataTypeStr=fixdt(1,14,9)
  Data Type Conversion1 : DataTypeConversion  OutDataTypeStr=double
  Data Type Conversion{9..11,15} (4 alike) : DataTypeConversion  OutDataTypeStr=fixdt(1,13,9)
  Data Type Conversion12 : DataTypeConversion  OutDataTypeStr=fixdt(1,3,0)
  Data Type Conversion13 : DataTypeConversion  OutDataTypeStr=fixdt(1,3,0)
  Data Type Conversion14 : DataTypeConversion  OutDataTypeStr=fixdt(1,4,0)
  Data Type Conversion16 : DataTypeConversion  OutDataTypeStr=fixdt(1,4,0)
  Data Type Conversion2 : DataTypeConversion  OutDataTypeStr=fixdt(1,14,9)
  Data Type Conversion3 : DataTypeConversion  OutDataTypeStr=double
  Data Type Conversion4 : DataTypeConversion  OutDataTypeStr=fixdt(1,14,9)
  Data Type Conversion5 : DataTypeConversion  OutDataTypeStr=double
  Data Type Conversion6 : DataTypeConversion  OutDataTypeStr=fixdt(1,2,0)
  Data Type Conversion7 : DataTypeConversion  OutDataTypeStr=fixdt(1,2,0)
  Data Type Conversion8 : DataTypeConversion  OutDataTypeStr=fixdt(1,2,0)
  Delay{,1,4..9} (8 alike) : Delay  DelayLength=1
  Delay2 : Delay  DelayLength=5
  Delay3 : Delay  DelayLength=3
  Gain : Gain  Gain=1/16
  Gain1 : Gain  Gain=4
  Sign : Signum
  Sign1 : Signum
  Sign2 : Signum
  Subtract : Sum  Inputs=+-
  Subtract1 : Sum  Inputs=+-
  Subtract2 : Sum  Inputs=+-
  Sum{,1..2,4,6} (5 alike) : Sum  Inputs=|++
  Sum3 : Sum  Inputs=|+-
  Sum5 : Sum  Inputs=|+-
  Out1 : Outport
  wires:
  Sum/1 -> Data Type Conversion/1
  Sum2/1 -> Data Type Conversion4/1
  Delay4/1 -> Sum2/2
  Delay8/1 -> Sum5/2
  Sum4/1 -> Data Type Conversion13/1
  Subtract/1 -> Data Type Conversion9/1
  Delay5/1 -> Sum3/1, Delay6/1
  Sign1/1 -> Data Type Conversion7/1
  Delay1/1 -> Sum1/2, Sum2/1
  Sum1/1 -> Data Type Conversion2/1
  Subtract1/1 -> Data Type Conversion10/1
  Sum3/1 -> Data Type Conversion12/1
  Delay/1 -> Sum/2, Sum1/1
  Delay3/1 -> Sum4/1
  Delay7/1 -> Sum4/2
  Subtract2/1 -> Data Type Conversion11/1
  Delay6/1 -> Sum3/2
  Sum5/1 -> Data Type Conversion14/1
  Delay2/1 -> Sum6/1
  Delay9/1 -> Sum6/2
  In1/1 -> Gain/1
  Sum6/1 -> Data Type Conversion16/1
  Data Type Conversion/1 -> Data Type Conversion1/1
  Data Type Conversion1/1 -> Subtract/1, Sign/1
  Data Type Conversion2/1 -> Data Type Conversion3/1
  Data Type Conversion4/1 -> Data Type Conversion5/1
  Data Type Conversion6/1 -> Subtract/2, Delay2/1
  Data Type Conversion7/1 -> Subtract1/2, Delay3/1
  Data Type Conversion8/1 -> Delay5/1, Subtract2/2
  Data Type Conversion9/1 -> Delay/1
  Data Type Conversion10/1 -> Delay1/1
  Data Type Conversion11/1 -> Delay4/1
  Data Type Conversion12/1 -> Delay7/1
  Data Type Conversion13/1 -> Sum5/1, Delay8/1
  Data Type Conversion14/1 -> Delay9/1
  Gain/1 -> Data Type Conversion15/1
  Gain1/1 -> Out1/1
  Data Type Conversion15/1 -> Sum/1
  Data Type Conversion16/1 -> Gain1/1
  Sign/1 -> Data Type Conversion6/1
  Data Type Conversion3/1 -> Sign1/1, Subtract1/1
  Data Type Conversion5/1 -> Sign2/1, Subtract2/1
  Sign2/1 -> Data Type Conversion8/1

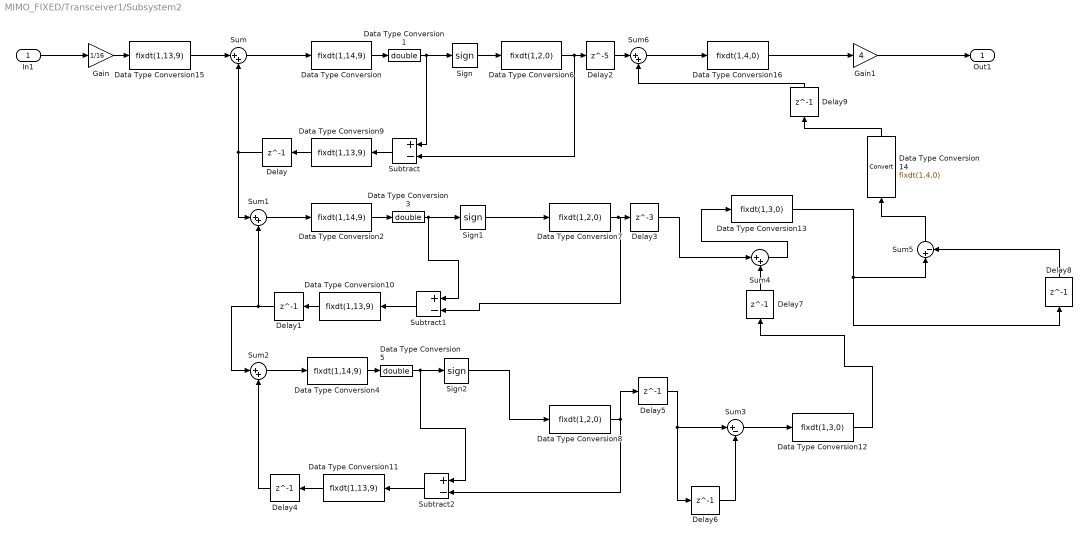
== system MIMO_FIXED/Transceiver1/Subsystem2 ==
  In1 : Inport
  Data Type Conversion : DataTypeConversion  OutDataTypeStr=fixdt(1,14,9)
  Data Type Conversion1 : DataTypeConversion  OutDataTypeStr=double
  Data Type Conversion{9..11,15} (4 alike) : DataTypeConversion  OutDataTypeStr=fixdt(1,13,9)
  Data Type Conversion12 : DataTypeConversion  OutDataTypeStr=fixdt(1,3,0)
  Data Type Conversion13 : DataTypeConversion  OutDataTypeStr=fixdt(1,3,0)
  Data Type Conversion14 : DataTypeConversion  OutDataTypeStr=fixdt(1,4,0)
  Data Type Conversion16 : DataTypeConversion  OutDataTypeStr=fixdt(1,4,0)
  Data Type Conversion2 : DataTypeConversion  OutDataTypeStr=fixdt(1,14,9)
  Data Type Conversion3 : DataTypeConversion  OutDataTypeStr=double
  Data Type Conversion4 : DataTypeConversion  OutDataTypeStr=fixdt(1,14,9)
  Data Type Conversion5 : DataTypeConversion  OutDataTypeStr=double
  Data Type Conversion6 : DataTypeConversion  OutDataTypeStr=fixdt(1,2,0)
  Data Type Conversion7 : DataTypeConversion  OutDataTypeStr=fixdt(1,2,0)
  Data Type Conversion8 : DataTypeConversion  OutDataTypeStr=fixdt(1,2,0)
  Delay{,1,4..9} (8 alike) : Delay  DelayLength=1
  Delay2 : Delay  DelayLength=5
  Delay3 : Delay  DelayLength=3
  Gain : Gain  Gain=1/16
  Gain1 : Gain  Gain=4
  Sign : Signum
  Sign1 : Signum
  Sign2 : Signum
  Subtract : Sum  Inputs=+-
  Subtract1 : Sum  Inputs=+-
  Subtract2 : Sum  Inputs=+-
  Sum{,1..2,4,6} (5 alike) : Sum  Inputs=|++
  Sum3 : Sum  Inputs=|+-
  Sum5 : Sum  Inputs=|+-
  Out1 : Outport
  wires:
  Sum/1 -> Data Type Conversion/1
  Sum2/1 -> Data Type Conversion4/1
  Delay4/1 -> Sum2/2
  Delay8/1 -> Sum5/2
  Sum4/1 -> Data Type Conversion13/1
  Subtract/1 -> Data Type Conversion9/1
  Delay5/1 -> Sum3/1, Delay6/1
  Sign1/1 -> Data Type Conversion7/1
  Delay1/1 -> Sum1/2, Sum2/1
  Sum1/1 -> Data Type Conversion2/1
  Subtract1/1 -> Data Type Conversion10/1
  Sum3/1 -> Data Type Conversion12/1
  Delay/1 -> Sum/2, Sum1/1
  Delay3/1 -> Sum4/1
  Delay7/1 -> Sum4/2
  Subtract2/1 -> Data Type Conversion11/1
  Delay6/1 -> Sum3/2
  Sum5/1 -> Data Type Conversion14/1
  Delay2/1 -> Sum6/1
  Delay9/1 -> Sum6/2
  In1/1 -> Gain/1
  Sum6/1 -> Data Type Conversion16/1
  Data Type Conversion/1 -> Data Type Conversion1/1
  Data Type Conversion1/1 -> Subtract/1, Sign/1
  Data Type Conversion2/1 -> Data Type Conversion3/1
  Data Type Conversion4/1 -> Data Type Conversion5/1
  Data Type Conversion6/1 -> Subtract/2, Delay2/1
  Data Type Conversion7/1 -> Subtract1/2, Delay3/1
  Data Type Conversion8/1 -> Delay5/1, Subtract2/2
  Data Type Conversion9/1 -> Delay/1
  Data Type Conversion10/1 -> Delay1/1
  Data Type Conversion11/1 -> Delay4/1
  Data Type Conversion12/1 -> Delay7/1
  Data Type Conversion13/1 -> Sum5/1, Delay8/1
  Data Type Conversion14/1 -> Delay9/1
  Gain/1 -> Data Type Conversion15/1
  Gain1/1 -> Out1/1
  Data Type Conversion15/1 -> Sum/1
  Data Type Conversion16/1 -> Gain1/1
  Sign/1 -> Data Type Conversion6/1
  Data Type Conversion3/1 -> Sign1/1, Subtract1/1
  Data Type Conversion5/1 -> Sign2/1, Subtract2/1
  Sign2/1 -> Data Type Conversion8/1

== system MIMO_FIXED/Transceiver5/ADC 1 ==
  In1 : Inport
  SigmaDelta ADC : Subsystem
  Switch : Switch  Criteria=u2 > Threshold  OutDataTypeStr=boolean
  Zero : Constant  Value=0
  bits 1&0 : Outport
  wires:
  SigmaDelta ADC/1(Out) -> Switch/1, Switch/2
  Zero/1 -> Switch/3
  In1/1 -> SigmaDelta ADC/1(In)
  Switch/1 -> bits 1&0/1

== system MIMO_FIXED/Transceiver5/CWM_RX2 ==
  In1 : Inport
  I_DDC : Inport  Port=2
  Q_DDC : Inport  Port=3
  Add : Sum
  Add1 : Sum  Inputs=-+
  Data Type Conversion{,1..9} (10 alike) : DataTypeConversion  OutDataTypeStr=fixdt(1,6,4)  SaturateOnIntegerOverflow=on
  Gain{,2,4,6} (4 alike) : Gain  Gain=-1
  Gain{1,3,5,7} (4 alike) : Gain
  Multiport Switch{,1,4..5} (4 alike) : MultiPortSwitch  DataPortOrder=Zero-based contiguous  Inputs=2  zeroidx=on  RndMeth=Nearest
  Trigonometric Function{,1,4..5} (4 alike) : Trigonometry
  Trigonometric Function{2..3,6..7} (4 alike) : Trigonometry  Operator=cos
  I` : Outport
  Q` : Outport  Port=2
  wires:
  Multiport Switch/1 -> Add1/1
  Add/1 -> Data Type Conversion8/1
  I_DDC/1 -> Multiport Switch1/1, Multiport Switch/1
  Gain2/1 -> Data Type Conversion6/1
  Trigonometric Function5/1 -> Gain5/1
  Data Type Conversion6/1 -> Multiport Switch1/2
  Data Type Conversion7/1 -> Multiport Switch/3
  Gain5/1 -> Data Type Conversion3/1
  Gain4/1 -> Data Type Conversion4/1
  Trigonometric Function1/1 -> Gain1/1
  Data Type Conversion2/1 -> Multiport Switch5/2
  Gain1/1 -> Data Type Conversion7/1
  Gain3/1 -> Data Type Conversion5/1
  Trigonometric Function3/1 -> Gain3/1
  Add1/1 -> Data Type Conversion9/1
  Gain/1 -> Data Type Conversion/1
  Trigonometric Function2/1 -> Gain2/1
  In1/1 -> Trigonometric Function3/1, Trigonometric Function6/1, Trigonometric Function7/1, Trigonometric Function5/1, Trigonometric Function4/1, Trigonometric Function2/1, Trigonometric Function1/1, Trigonometric Function/1
  Q_DDC/1 -> Multiport Switch5/1, Multiport Switch4/1
  Data Type Conversion1/1 -> Multiport Switch5/3
  Data Type Conversion4/1 -> Multiport Switch4/2
  Trigonometric Function6/1 -> Gain6/1
  Gain7/1 -> Data Type Conversion1/1
  Trigonometric Function4/1 -> Gain4/1
  Trigonometric Function/1 -> Gain/1
  Multiport Switch1/1 -> Add/1
  Multiport Switch4/1 -> Add/2
  Trigonometric Function7/1 -> Gain7/1
  Multiport Switch5/1 -> Add1/2
  Data Type Conversion3/1 -> Multiport Switch4/3
  Gain6/1 -> Data Type Conversion2/1
  Data Type Conversion/1 -> Multiport Switch/2
  Data Type Conversion5/1 -> Multiport Switch1/3
  Data Type Conversion8/1 -> I`/1
  Data Type Conversion9/1 -> Q`/1

== system MIMO_FIXED/Transceiver5/CWM_TX_Chain_1 ==
  PHI : Inport
  Processor_I : Inport  Port=2
  Processor_Q : Inport  Port=3
  Add : Sum  OutDataTypeStr=double  RndMeth=Round  SaturateOnIntegerOverflow=on
  Add1 : Sum  OutDataTypeStr=double
  Data Type Conversion : DataTypeConversion  OutDataTypeStr=fixdt(1,6,4)  SaturateOnIntegerOverflow=on
  Data Type Conversion1 : DataTypeConversion  OutDataTypeStr=fixdt(1,6,4)  RndMeth=Round  SaturateOnIntegerOverflow=on
  Data Type Conversion12 : DataTypeConversion  OutDataTypeStr=fixdt(1,16,9)  SaturateOnIntegerOverflow=on
  Data Type Conversion2 : DataTypeConversion  OutDataTypeStr=fixdt(1,6,4)  RndMeth=Round  SaturateOnIntegerOverflow=on
  Data Type Conversion3 : DataTypeConversion  OutDataTypeStr=fixdt(1,6,4)  SaturateOnIntegerOverflow=on
  Data Type Conversion4 : DataTypeConversion  OutDataTypeStr=fixdt(1,16,7)  SaturateOnIntegerOverflow=on
  Data Type Conversion5 : DataTypeConversion  OutDataTypeStr=fixdt(1,16,9)  SaturateOnIntegerOverflow=on
  Data Type Conversion6 : DataTypeConversion  OutDataTypeStr=fixdt(1,16,9)  SaturateOnIntegerOverflow=on
  Data Type Conversion7 : DataTypeConversion  OutDataTypeStr=fixdt(1,18,9)  SaturateOnIntegerOverflow=on
  Data Type Conversion8 : DataTypeConversion  OutDataTypeStr=fixdt(1,18,9)  SaturateOnIntegerOverflow=on
  Gain1 : Gain  Gain=-1
  Gain2 : Gain
  Gain3 : Gain
  Gain4 : Gain
  Product{,1..3} (4 alike) : Product
  Trigonometric Function1 : Trigonometry
  Trigonometric Function2 : Trigonometry  Operator=cos
  Trigonometric Function3 : Trigonometry  Operator=cos
  Trigonometric Function4 : Trigonometry
  I_1 : Outport
  Q_1 : Outport  Port=2
  wires:
  Trigonometric Function2/1 -> Gain2/1
  Gain2/1 -> Data Type Conversion/1
  Processor_Q/1 -> Product1/2, Product3/2
  Processor_I/1 -> Product2/1, Product/1
  Gain1/1 -> Data Type Conversion1/1
  Product/1 -> Data Type Conversion12/1
  Trigonometric Function1/1 -> Gain1/1
  PHI/1 -> Trigonometric Function2/1, Trigonometric Function1/1, Trigonometric Function4/1, Trigonometric Function3/1
  Data Type Conversion1/1 -> Product1/1
  Gain3/1 -> Data Type Conversion3/1
  Product2/1 -> Data Type Conversion5/1
  Data Type Conversion/1 -> Product/2
  Data Type Conversion2/1 -> Product2/2
  Data Type Conversion3/1 -> Product3/1
  Product3/1 -> Data Type Conversion6/1
  Trigonometric Function3/1 -> Gain3/1
  Product1/1 -> Data Type Conversion4/1
  Gain4/1 -> Data Type Conversion2/1
  Trigonometric Function4/1 -> Gain4/1
  Add1/1 -> Data Type Conversion8/1
  Data Type Conversion7/1 -> I_1/1
  Data Type Conversion8/1 -> Q_1/1
  Data Type Conversion12/1 -> Add/1
  Data Type Conversion4/1 -> Add/2
  Data Type Conversion5/1 -> Add1/1
  Data Type Conversion6/1 -> Add1/2
  Add/1 -> Data Type Conversion7/1

== system MIMO_FIXED/Transceiver5/DDC2 ==
  ODD_I : Inport
  EVEN_Q : Inport  Port=2
  Local_Oscilator1 : DiscretePulseGenerator  PhaseDelay=1  SampleTime=0.02
  Logical Operator : Logic  Operator=NXOR  AllPortsSameDT=off  OutDataTypeStr=boolean
  Logical Operator1 : Logic  Operator=NXOR  AllPortsSameDT=off  OutDataTypeStr=boolean
  NOT : Logic  Operator=NOT  IconShape=distinctive  AllPortsSameDT=off  OutDataTypeStr=boolean
  I_DDC : Outport
  Q_DDC : Outport  Port=2
  wires:
  Logical Operator/1 -> I_DDC/1
  EVEN_Q/1 -> Logical Operator1/2
  ODD_I/1 -> Logical Operator/1
  Logical Operator1/1 -> Q_DDC/1
  Local_Oscilator1/1 -> NOT/1
  NOT/1 -> Logical Operator1/1, Logical Operator/2

== system MIMO_FIXED/Transceiver5/DUC2 ==
  I_1 : Inport
  Q_1 : Inport  Port=2
  -cos : Sin  SineType=Sample based  Frequency=2*pi*100  Phase=pi/2  Samples=4  SampleTime=0.01  Offset=3
  -sin1 : Sin  SineType=Sample based  Frequency=(2*pi*100)/4  Samples=4  SampleTime=.01  Offset=2
  Add : Sum
  Constant : Constant  Value=0
  Constant1 : Constant  Value=0
  Data Type Conversion : DataTypeConversion  OutDataTypeStr=fixdt(1,2,0)  RndMeth=Round
  Data Type Conversion1 : DataTypeConversion  OutDataTypeStr=fixdt(1,2,0)  RndMeth=Round
  Data Type Conversion{2..3,5..6} (4 alike) : DataTypeConversion  OutDataTypeStr=fixdt(1,6,0)
  Data Type Conversion4 : DataTypeConversion  OutDataTypeStr=fixdt(1,7,0)
  Gain : Gain  Gain=-1
  Gain1 : Gain  Gain=-1
  Multiport Switch : MultiPortSwitch  DataPortOrder=Specify indices  DataPortIndices={1,0,-1}  RndMeth=Nearest
  Multiport Switch1 : MultiPortSwitch  DataPortOrder=Specify indices  DataPortIndices={1,0,-1}  RndMeth=Nearest
  Out2 : Outport
  wires:
  Constant/1 -> Multiport Switch1/3
  Q_1/1 -> Multiport Switch/2, Gain1/1
  I_1/1 -> Multiport Switch1/2, Gain/1
  Gain1/1 -> Data Type Conversion2/1
  -sin1/1 -> Data Type Conversion1/1
  -cos/1 -> Data Type Conversion/1
  Multiport Switch/1 -> Data Type Conversion5/1
  Add/1 -> Data Type Conversion4/1
  Multiport Switch1/1 -> Data Type Conversion6/1
  Constant1/1 -> Multiport Switch/3
  Gain/1 -> Data Type Conversion3/1
  Data Type Conversion/1 -> Multiport Switch1/1
  Data Type Conversion1/1 -> Multiport Switch/1
  Data Type Conversion2/1 -> Multiport Switch/4
  Data Type Conversion3/1 -> Multiport Switch1/4
  Data Type Conversion6/1 -> Add/1
  Data Type Conversion5/1 -> Add/2
  Data Type Conversion4/1 -> Out2/1

== system MIMO_FIXED/Transceiver5/Inter_Lever2 ==
  bits 1&0 : Inport
  Delay1 : Delay  DelayLength=1  InitialCondition=0
  Delay2 : Delay  DelayLength=1  InitialCondition=0
  Downsample : DownSample  RateOptions=Allow multirate processing
  Downsample1 : DownSample  RateOptions=Allow multirate processing
  ODD_I : Outport
  EVEN_Q : Outport  Port=2
  wires:
  Delay1/1 -> Downsample1/1
  Downsample/1 -> Delay2/1
  Downsample1/1 -> EVEN_Q/1
  bits 1&0/1 -> Delay1/1, Downsample/1
  Delay2/1 -> ODD_I/1

== system MIMO_FIXED/Transceiver5/Interpolation 1 ==
  Input : Inport
  Data Type Conversion2 : DataTypeConversion  OutDataTypeStr=fixdt(1,11,6)  SaturateOnIntegerOverflow=on
  Data Type Conversion5 : DataTypeConversion  OutDataTypeStr=fixdt(1,23,0)  SaturateOnIntegerOverflow=on
  Gain : Gain  Gain=512
  Gain1 : Gain  Gain=1/64
  Gain2 : Gain  Gain=1/512
  Gain3 : Gain  Gain=1/512
  Gain5 : Gain  Gain=64
  Half_band : Subsystem
  comb_filter : Subsystem
  Out1 : Outport
  wires:
  Input/1 -> Gain/1
  Gain5/1 -> comb_filter/1(In1)
  Gain1/1 -> Out1/1
  Data Type Conversion2/1 -> Gain5/1
  Gain2/1 -> Gain3/1
  Gain3/1 -> Data Type Conversion2/1
  Data Type Conversion5/1 -> Gain2/1
  Gain/1 -> Half_band/1(Input)
  Half_band/1(Out1) -> Data Type Conversion5/1
  comb_filter/1(Out1) -> Gain1/1
